simulink model "lab3"  (R2024a)
settings: Solver=VariableStepAuto  StartTime=0.0  StopTime=20.0  RelTol=1e-3
libraries: cstblocks x4
settings Model: Creator=PMYLS  LastModifiedBy=PMYLS

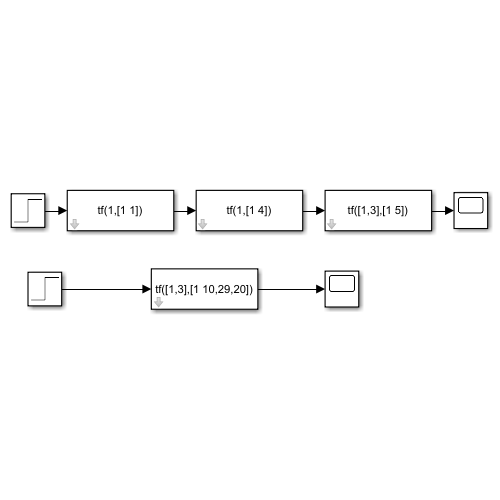
[thumbnail: Simulink's stored preview of the top-level diagram]
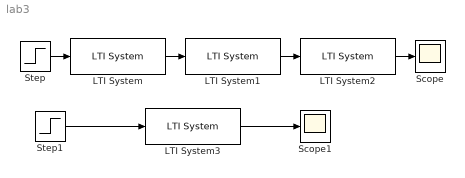
== system lab3 ==
  LTI System : cstblocks/LTI System  sys=tf(1,[1 1])  IC=[]  PadeOrder=0
  LTI System1 : cstblocks/LTI System  sys=tf(1,[1 4])  IC=[]  PadeOrder=0
  LTI System2 : cstblocks/LTI System  sys=tf([1,3],[1 5])  IC=[]  PadeOrder=0
  LTI System3 : cstblocks/LTI System  sys=tf([1,3],[1 10,29,20])  IC=[]  PadeOrder=0
  Scope : Scope
  Scope1 : Scope
  Step : Step  SampleTime=0
  Step1 : Step  SampleTime=0
  wires:
  LTI System/1 -> LTI System1/1
  LTI System1/1 -> LTI System2/1
  Step/1 -> LTI System/1
  LTI System2/1 -> Scope/1
  Step1/1 -> LTI System3/1
  LTI System3/1 -> Scope1/1
